simulink model "tpd97a1049_9da9_400b_b646_69a6eb2b8ed0"  (R2026a)
settings: Solver=ode45  StartTime=0  StopTime=1  MaxStep=5.0000000000000002e-05  RelTol=9.9999999999999995e-08  AbsTol=1.0000000000000001e-09
model workspace (MAT data in the model file):
  mc.model = 'MotionCore'
  mc.motor.Ra = 2
  mc.motor.La = 0.002
  mc.motor.Ke = 0.05
  mc.motor.Kt = 0.05
  mc.motor.J = 0.0001
  mc.motor.b = 0.0001
  mc.initial.current_A = 0
  mc.initial.omega_rad_s = 0
  mc.input.step_time_s = 0.05
  mc.input.voltage_before_V = 0
  mc.input.voltage_after_V = 12
  mc.input.load_torque_Nm = 0
  mc.units.rad_s_to_rpm = 9.54929658551
  mc.sim.stop_time_s = 0.8
  mc.sim.solver = 'ode45'
  mc.sim.max_step_s = 5e-05
  mc.sim.rel_tol = 1e-07
  mc.sim.abs_tol = 1e-09
  mc.check.state_relative_tol = 0.0001
  mc.check.steady_relative_tol = 0.002
  mc.check.energy_relative_tol = 0.005
  mc.math.A = [-1000  -25; 500  -1]
  mc.math.B = [500  0; 0  -10000]
  mc.math.C = [1  0; 0  1]
  mc.math.D = [0  0; 0  0]
  mc.math.speed_tf_num = 0.05
  mc.math.speed_tf_den = [2e-07 0.0002002 0.0027]
  mc.math.poles = [-987.32671455; -13.6732854495]
  mc.math.slow_tau_s = 0.0731353121889
  mc.math.electrical_tau_s = 0.001
  mc.math.final_state = [0.444444444444; 222.222222222]
  p3.model = 'MotionCore_Phase3'
  p3.Ts = 0.001
  p3.bandwidth_rad_s = 15
  p3.candidate_bandwidths = [8 15 25]
  p3.test_speeds_rpm = [500 1000 1500 2000]
  p3.step_time_s = 0.05
  p3.stop_time_s = 1
  p3.reference_rpm = 1000
  p3.initial_reference_rpm = 0
  p3.second_step_s = 0.65
  p3.second_step_delta_rpm = 0
  p3.voltage_min_V = 0
  p3.voltage_max_V = 12
  p3.Kd = 0
  p3.derivative_filter_s = 0.005
  p3.antiwindup_time_s = 0.05
  p3.Kb = 20
  p3.integrator_initial_V = 0
  p3.load_Nm = 0
  p3.check.steady_error_rpm = 1
  p3.check.settling_band_fraction = 0.02
  p3.check.settling_limit_s = 0.5
  p3.check.hold_time_s = 0.05
  p3.check.overshoot_limit_pct = 5
  p3.check.reference_relative_tol = 0.0002
  p3.check.identity_relative_tol = 1e-07
  p3.check.energy_relative_tol = 0.005
  p3.A = [-1000  -25; 500  -1]
  p3.B = [500  0; 0  -10000]
  p3.slow_pole_rad_s = 13.6732854495
  p3.fast_pole_rad_s = 987.32671455
  p3.dc_gain_rpm_V = 176.838825658
  p3.Kp = 0.00620355670625
  p3.Ki = 0.0848230016469
  p3.derivative_a = 0.833333333333
  p3.derivative_b = 166.666666667
  p4.model = 'MotionCore_Phase4'
  p4.phase3_model = 'MotionCore_Phase3'
  p4.controller_Ts = 0.001
  p4.Ts = 0.001
  p4.Kp = 0.00620355670625
  p4.Ki = 0.0848230016469
  p4.Kd = 0
  p4.Kb = 20
  p4.fpwm_Hz = 20000
  p4.Tpwm_s = 5e-05
  p4.controller_frequency_Hz = 1000
  p4.Vdc_V = 12
  p4.PWM_BITS = 12
  p4.quantized_duty_experiment = 0
  p4.test_speeds_rpm = [500 1000 1500 2000]
  p4.reference_rpm = 1000
  p4.initial_reference_rpm = 0
  p4.step_time_s = 0.05
  p4.stop_time_s = 1
  p4.load_Nm = 0
  p4.second_step_s = 0.65
  p4.second_step_delta_rpm = 0
  p4.voltage_min_V = 0
  p4.voltage_max_V = 12
  p4.antiwindup_time_s = 0.05
  p4.check.steady_error_rpm = 1
  p4.check.settling_band_fraction = 0.02
  p4.check.settling_limit_s = 0.5
  p4.check.hold_time_s = 0.05
  p4.check.overshoot_limit_pct = 5
  p4.check.reference_relative_tol = 0.0002
  p4.check.identity_relative_tol = 1e-07
  p4.check.energy_relative_tol = 0.005
  p4.check.phase3_regression_relative_tol = 2e-06
  p4.check.pwm_identity_relative_tol = 2e-08
  p4.check.duty_tolerance = 2e-08
  p4.check.max_phase3_regression_abs_rpm = 0.001
  p4.check.max_phase3_regression_abs_current_A = 1e-06
settings Model: Creator=peizh  LastModifiedBy=peizh

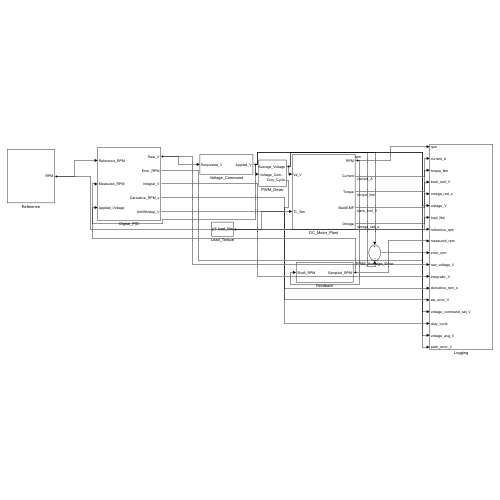
[thumbnail: Simulink's stored preview of the top-level diagram]
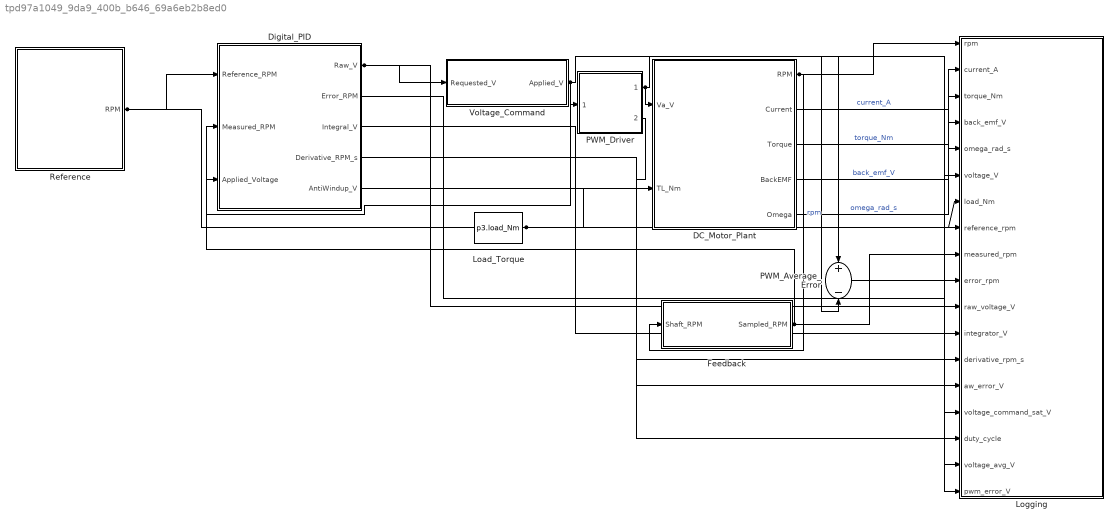
== system tpd97a1049_9da9_400b_b646_69a6eb2b8ed0 ==
  DC_Motor_Plant : Subsystem
  Digital_PID : Subsystem
  Feedback : Subsystem
  Load_Torque : Constant  Value=p3.load_Nm
  Logging : Subsystem
  PWM_Average_Error : Sum  Inputs=+-
  PWM_Driver : Subsystem
  Reference : Subsystem
  Voltage_Command : Subsystem
  wires:
  Reference/1(RPM) -> Digital_PID/1(Reference_RPM), Logging/8(reference_rpm)
  Feedback/1(Sampled_RPM) -> Digital_PID/2(Measured_RPM), Logging/9(measured_rpm)
  Digital_PID/1(Raw_V) -> Voltage_Command/1(Requested_V), Logging/11(raw_voltage_V)
  Voltage_Command/1(Applied_V) -> Digital_PID/3(Applied_Voltage), PWM_Driver/1(Voltage_Command_Sat), Logging/6(voltage_V), PWM_Average_Error/2, Logging/15(voltage_command_sat_V)
  PWM_Driver/1(Average_Voltage) -> DC_Motor_Plant/1(Va_V), PWM_Average_Error/1, Logging/17(voltage_avg_V)
  Load_Torque/1 -> DC_Motor_Plant/2(TL_Nm), Logging/7(load_Nm)
  DC_Motor_Plant/1(RPM) -> Feedback/1(Shaft_RPM), Logging/1(rpm)  "rpm"
  DC_Motor_Plant/2(Current) -> Logging/2(current_A)  "current_A"
  DC_Motor_Plant/3(Torque) -> Logging/3(torque_Nm)  "torque_Nm"
  DC_Motor_Plant/4(BackEMF) -> Logging/4(back_emf_V)  "back_emf_V"
  DC_Motor_Plant/5(Omega) -> Logging/5(omega_rad_s)  "omega_rad_s"
  Digital_PID/2(Error_RPM) -> Logging/10(error_rpm)
  Digital_PID/3(Integral_V) -> Logging/12(integrator_V)
  Digital_PID/4(Derivative_RPM_s) -> Logging/13(derivative_rpm_s)
  Digital_PID/5(AntiWindup_V) -> Logging/14(aw_error_V)
  PWM_Driver/2(Duty_Cycle) -> Logging/16(duty_cycle)
  PWM_Average_Error/1 -> Logging/18(pwm_error_V)

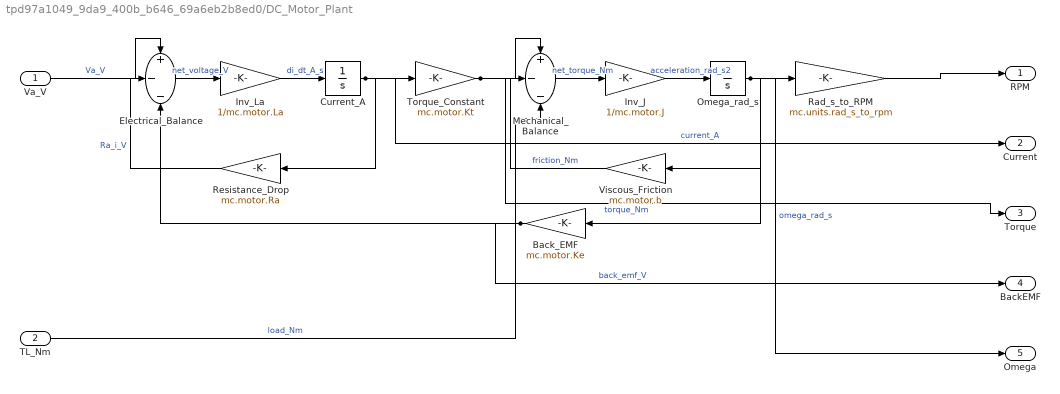
== system tpd97a1049_9da9_400b_b646_69a6eb2b8ed0/DC_Motor_Plant ==
  Va_V : Inport
  TL_Nm : Inport  Port=2
  Back_EMF : Gain  Gain=mc.motor.Ke
  Current_A : Integrator  InitialCondition=mc.initial.current_A
  Electrical_Balance : Sum  Inputs=+--
  Inv_J : Gain  Gain=1/mc.motor.J
  Inv_La : Gain  Gain=1/mc.motor.La
  Mechanical_Balance : Sum  Inputs=+--
  Omega_rad_s : Integrator  InitialCondition=mc.initial.omega_rad_s
  Rad_s_to_RPM : Gain  Gain=mc.units.rad_s_to_rpm
  Resistance_Drop : Gain  Gain=mc.motor.Ra
  Torque_Constant : Gain  Gain=mc.motor.Kt
  Viscous_Friction : Gain  Gain=mc.motor.b
  RPM : Outport
  Current : Outport  Port=2
  Torque : Outport  Port=3
  BackEMF : Outport  Port=4
  Omega : Outport  Port=5
  wires:
  Va_V/1 -> Electrical_Balance/1  "Va_V"
  Electrical_Balance/1 -> Inv_La/1  "net_voltage_V"
  Inv_La/1 -> Current_A/1  "di_dt_A_s"
  Current_A/1 -> Resistance_Drop/1, Torque_Constant/1, Current/1  "current_A"
  Resistance_Drop/1 -> Electrical_Balance/2  "Ra_i_V"
  Torque_Constant/1 -> Mechanical_Balance/1, Torque/1  "torque_Nm"
  Viscous_Friction/1 -> Mechanical_Balance/2  "friction_Nm"
  TL_Nm/1 -> Mechanical_Balance/3  "load_Nm"
  Mechanical_Balance/1 -> Inv_J/1  "net_torque_Nm"
  Inv_J/1 -> Omega_rad_s/1  "acceleration_rad_s2"
  Omega_rad_s/1 -> Viscous_Friction/1, Back_EMF/1, Rad_s_to_RPM/1, Omega/1  "omega_rad_s"
  Back_EMF/1 -> Electrical_Balance/3, BackEMF/1  "back_emf_V"
  Rad_s_to_RPM/1 -> RPM/1

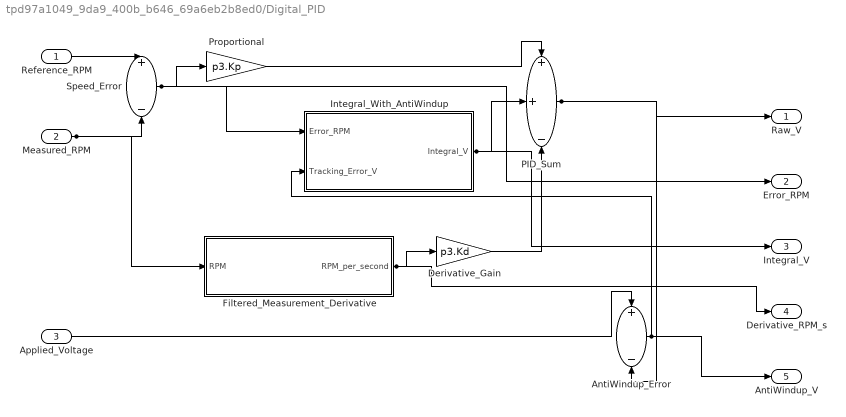
== system tpd97a1049_9da9_400b_b646_69a6eb2b8ed0/Digital_PID ==
  Reference_RPM : Inport
  Measured_RPM : Inport  Port=2
  Applied_Voltage : Inport  Port=3
  AntiWindup_Error : Sum  Inputs=+-
  Derivative_Gain : Gain  Gain=p3.Kd
  Filtered_Measurement_Derivative : Subsystem
  Integral_With_AntiWindup : Subsystem
  PID_Sum : Sum  Inputs=++-
  Proportional : Gain  Gain=p3.Kp
  Speed_Error : Sum  Inputs=+-
  Raw_V : Outport
  Error_RPM : Outport  Port=2
  Integral_V : Outport  Port=3
  Derivative_RPM_s : Outport  Port=4
  AntiWindup_V : Outport  Port=5
  wires:
  Derivative_Gain/1 -> PID_Sum/3
  Filtered_Measurement_Derivative/1(RPM_per_second) -> Derivative_RPM_s/1, Derivative_Gain/1
  Integral_With_AntiWindup/1(Integral_V) -> Integral_V/1, PID_Sum/2
  AntiWindup_Error/1 -> AntiWindup_V/1, Integral_With_AntiWindup/2(Tracking_Error_V)
  PID_Sum/1 -> Raw_V/1, AntiWindup_Error/2
  Applied_Voltage/1 -> AntiWindup_Error/1
  Proportional/1 -> PID_Sum/1
  Speed_Error/1 -> Error_RPM/1, Integral_With_AntiWindup/1(Error_RPM), Proportional/1
  Measured_RPM/1 -> Filtered_Measurement_Derivative/1(RPM), Speed_Error/2
  Reference_RPM/1 -> Speed_Error/1

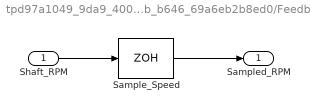
== system tpd97a1049_9da9_400b_b646_69a6eb2b8ed0/Feedback ==
  Shaft_RPM : Inport
  Sample_Speed : ZeroOrderHold  SampleTime=p3.Ts
  Sampled_RPM : Outport
  wires:
  Sample_Speed/1 -> Sampled_RPM/1
  Shaft_RPM/1 -> Sample_Speed/1

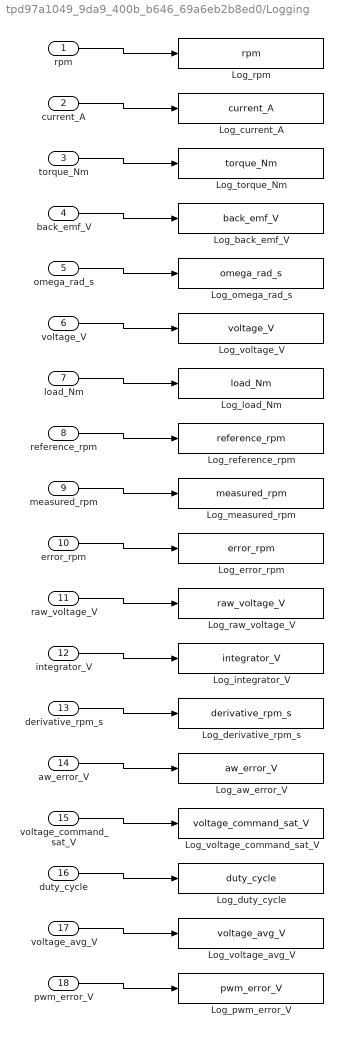
== system tpd97a1049_9da9_400b_b646_69a6eb2b8ed0/Logging ==
  rpm : Inport
  current_A : Inport  Port=2
  torque_Nm : Inport  Port=3
  back_emf_V : Inport  Port=4
  omega_rad_s : Inport  Port=5
  voltage_V : Inport  Port=6
  load_Nm : Inport  Port=7
  reference_rpm : Inport  Port=8
  measured_rpm : Inport  Port=9
  error_rpm : Inport  Port=10
  raw_voltage_V : Inport  Port=11
  integrator_V : Inport  Port=12
  derivative_rpm_s : Inport  Port=13
  aw_error_V : Inport  Port=14
  voltage_command_sat_V : Inport  Port=15
  duty_cycle : Inport  Port=16
  voltage_avg_V : Inport  Port=17
  pwm_error_V : Inport  Port=18
  Log_aw_error_V : ToWorkspace  VariableName=aw_error_V  SaveFormat=Timeseries  SampleTime=-1
  Log_back_emf_V : ToWorkspace  VariableName=back_emf_V  SaveFormat=Timeseries  SampleTime=-1
  Log_current_A : ToWorkspace  VariableName=current_A  SaveFormat=Timeseries  SampleTime=-1
  Log_derivative_rpm_s : ToWorkspace  VariableName=derivative_rpm_s  SaveFormat=Timeseries  SampleTime=-1
  Log_duty_cycle : ToWorkspace  VariableName=duty_cycle  SaveFormat=Timeseries  SampleTime=-1
  Log_error_rpm : ToWorkspace  VariableName=error_rpm  SaveFormat=Timeseries  SampleTime=-1
  Log_integrator_V : ToWorkspace  VariableName=integrator_V  SaveFormat=Timeseries  SampleTime=-1
  Log_load_Nm : ToWorkspace  VariableName=load_Nm  SaveFormat=Timeseries  SampleTime=-1
  Log_measured_rpm : ToWorkspace  VariableName=measured_rpm  SaveFormat=Timeseries  SampleTime=-1
  Log_omega_rad_s : ToWorkspace  VariableName=omega_rad_s  SaveFormat=Timeseries  SampleTime=-1
  Log_pwm_error_V : ToWorkspace  VariableName=pwm_error_V  SaveFormat=Timeseries  SampleTime=-1
  Log_raw_voltage_V : ToWorkspace  VariableName=raw_voltage_V  SaveFormat=Timeseries  SampleTime=-1
  Log_reference_rpm : ToWorkspace  VariableName=reference_rpm  SaveFormat=Timeseries  SampleTime=-1
  Log_rpm : ToWorkspace  VariableName=rpm  SaveFormat=Timeseries  SampleTime=-1
  Log_torque_Nm : ToWorkspace  VariableName=torque_Nm  SaveFormat=Timeseries  SampleTime=-1
  Log_voltage_V : ToWorkspace  VariableName=voltage_V  SaveFormat=Timeseries  SampleTime=-1
  Log_voltage_avg_V : ToWorkspace  VariableName=voltage_avg_V  SaveFormat=Timeseries  SampleTime=-1
  Log_voltage_command_sat_V : ToWorkspace  VariableName=voltage_command_sat_V  SaveFormat=Timeseries  SampleTime=-1
  wires:
  aw_error_V/1 -> Log_aw_error_V/1
  derivative_rpm_s/1 -> Log_derivative_rpm_s/1
  integrator_V/1 -> Log_integrator_V/1
  raw_voltage_V/1 -> Log_raw_voltage_V/1
  error_rpm/1 -> Log_error_rpm/1
  measured_rpm/1 -> Log_measured_rpm/1
  reference_rpm/1 -> Log_reference_rpm/1
  load_Nm/1 -> Log_load_Nm/1
  voltage_V/1 -> Log_voltage_V/1
  omega_rad_s/1 -> Log_omega_rad_s/1
  back_emf_V/1 -> Log_back_emf_V/1
  torque_Nm/1 -> Log_torque_Nm/1
  current_A/1 -> Log_current_A/1
  rpm/1 -> Log_rpm/1
  voltage_command_sat_V/1 -> Log_voltage_command_sat_V/1
  duty_cycle/1 -> Log_duty_cycle/1
  voltage_avg_V/1 -> Log_voltage_avg_V/1
  pwm_error_V/1 -> Log_pwm_error_V/1

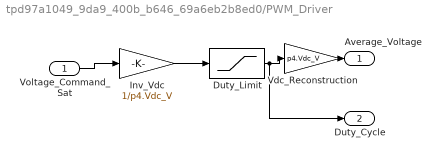
== system tpd97a1049_9da9_400b_b646_69a6eb2b8ed0/PWM_Driver ==
  Voltage_Command_Sat : Inport
  Duty_Limit : Saturate  UpperLimit=1  LowerLimit=0
  Inv_Vdc : Gain  Gain=1/p4.Vdc_V
  Vdc_Reconstruction : Gain  Gain=p4.Vdc_V
  Average_Voltage : Outport
  Duty_Cycle : Outport  Port=2
  wires:
  Voltage_Command_Sat/1 -> Inv_Vdc/1
  Inv_Vdc/1 -> Duty_Limit/1
  Duty_Limit/1 -> Vdc_Reconstruction/1, Duty_Cycle/1
  Vdc_Reconstruction/1 -> Average_Voltage/1

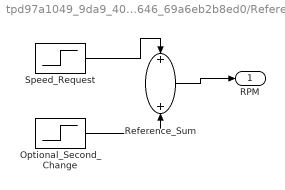
== system tpd97a1049_9da9_400b_b646_69a6eb2b8ed0/Reference ==
  Optional_Second_Change : Step  Time=p3.second_step_s  FinalValue=p3.second_step_delta_rpm  SampleTime=p3.Ts
  Reference_Sum : Sum
  Speed_Request : Step  Time=p3.step_time_s  InitialValue=p3.initial_reference_rpm  FinalValue=p3.reference_rpm  SampleTime=p3.Ts
  RPM : Outport
  wires:
  Reference_Sum/1 -> RPM/1
  Optional_Second_Change/1 -> Reference_Sum/2
  Speed_Request/1 -> Reference_Sum/1

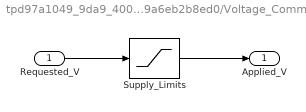
== system tpd97a1049_9da9_400b_b646_69a6eb2b8ed0/Voltage_Command ==
  Requested_V : Inport
  Supply_Limits : Saturate  UpperLimit=p3.voltage_max_V  LowerLimit=p3.voltage_min_V
  Applied_V : Outport
  wires:
  Supply_Limits/1 -> Applied_V/1
  Requested_V/1 -> Supply_Limits/1

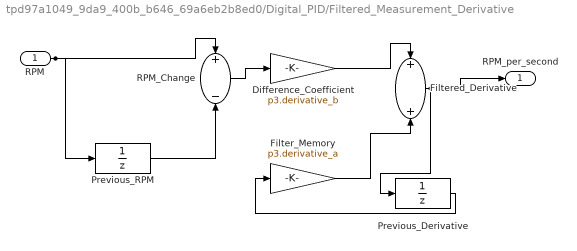
== system tpd97a1049_9da9_400b_b646_69a6eb2b8ed0/Digital_PID/Filtered_Measurement_Derivative ==
  RPM : Inport
  Difference_Coefficient : Gain  Gain=p3.derivative_b
  Filter_Memory : Gain  Gain=p3.derivative_a
  Filtered_Derivative : Sum
  Previous_Derivative : UnitDelay  SampleTime=p3.Ts
  Previous_RPM : UnitDelay  InitialCondition=mc.initial.omega_rad_s*mc.units.rad_s_to_rpm  SampleTime=p3.Ts
  RPM_Change : Sum  Inputs=+-
  RPM_per_second : Outport
  wires:
  Filter_Memory/1 -> Filtered_Derivative/2
  Previous_Derivative/1 -> Filter_Memory/1
  Filtered_Derivative/1 -> RPM_per_second/1, Previous_Derivative/1
  Difference_Coefficient/1 -> Filtered_Derivative/1
  RPM_Change/1 -> Difference_Coefficient/1
  Previous_RPM/1 -> RPM_Change/2
  RPM/1 -> Previous_RPM/1, RPM_Change/1

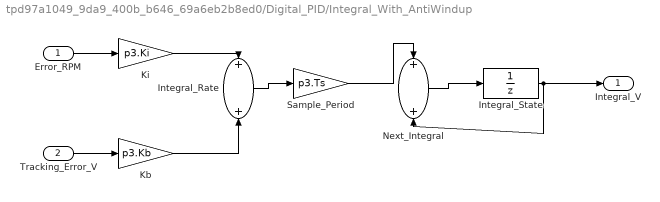
== system tpd97a1049_9da9_400b_b646_69a6eb2b8ed0/Digital_PID/Integral_With_AntiWindup ==
  Error_RPM : Inport
  Tracking_Error_V : Inport  Port=2
  Integral_Rate : Sum
  Integral_State : UnitDelay  InitialCondition=p3.integrator_initial_V  SampleTime=p3.Ts
  Kb : Gain  Gain=p3.Kb
  Ki : Gain  Gain=p3.Ki
  Next_Integral : Sum
  Sample_Period : Gain  Gain=p3.Ts
  Integral_V : Outport
  wires:
  Next_Integral/1 -> Integral_State/1
  Integral_State/1 -> Integral_V/1, Next_Integral/2
  Sample_Period/1 -> Next_Integral/1
  Integral_Rate/1 -> Sample_Period/1
  Kb/1 -> Integral_Rate/2
  Ki/1 -> Integral_Rate/1
  Tracking_Error_V/1 -> Kb/1
  Error_RPM/1 -> Ki/1
